simulink model "I_Control_Dcmotor"  (R2022b)
settings: Solver=ode4  StartTime=0.0  StopTime=inf  RelTol=1e-3  EnableMultiTasking=on
libraries: arduinolib x4, arduinosensorlib x1
settings Model: ExtModeTrigDuration=2  Creator=user  LastModifiedBy=user
settings OptimizationCC: EnhancedBackFolding=on  PassReuseOutputArgsAs=Individual arguments  ZeroExternalMemoryAtStartup=off  ZeroInternalMemoryAtStartup=off  MaxStackSize=64  OptimizeBlockOrder=speed  DifferentSizesBufferReuse=on  OptimizationCustomize=off  EfficientTunableParamExpr=on
settings DebuggingCC: ParameterTunabilityLossMsg=error
settings HardwareCC: ProdBitPerInt=16  ProdBitPerPointer=16  ProdBitPerSizeT=16  ProdBitPerPtrDiffT=16  ProdLargestAtomicFloat=None  ProdWordSize=8  ProdHWDeviceType=Atmel->AVR
settings SFSimCC: MATLABDynamicMemAlloc=off
settings RTWCC: Description=Embedded Coder  SystemTargetFile=ert.tlc  HardwareBoard=Arduino Mega 2560  TLCOptions=-aInlineSetEventsForThisBaseRateFcn=TLC_FALSE -aSuppressMultiTaskScheduler=TLC_FALSE -aRateBasedStepFcn=1  TemplateMakefile=ert_default_tmf  Toolchain=Arduino AVR  BuildConfiguration=Faster Runs
settings CodeAppCC: ForceParamTrailComments=on  IgnoreCustomStorageClasses=off  OperatorAnnotations=on  SimulinkDataObjDesc=on  SFDataObjDesc=on  InsertBlockDesc=on
settings ERTTargetCC: SupportContinuousTime=on  SupportVariableSizeSignals=on  ExtModeTransport=3  ExtModeStaticAlloc=on  ExtModeAutomaticAllocSize=off  ExtModeStaticAllocSize=2048  ExtModeMexFile=ext_xcp  ExtModeIntrfLevel=Level2 - Open

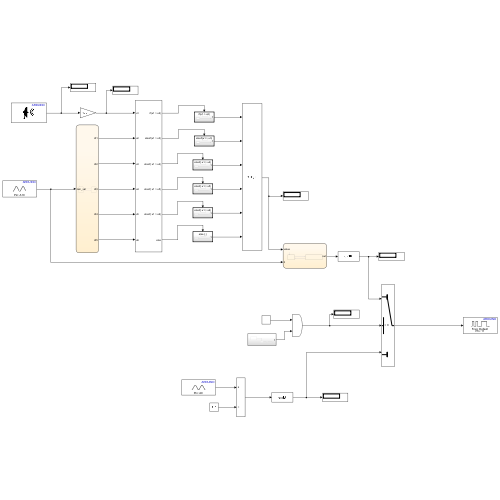
[thumbnail: Simulink's stored preview of the top-level diagram]
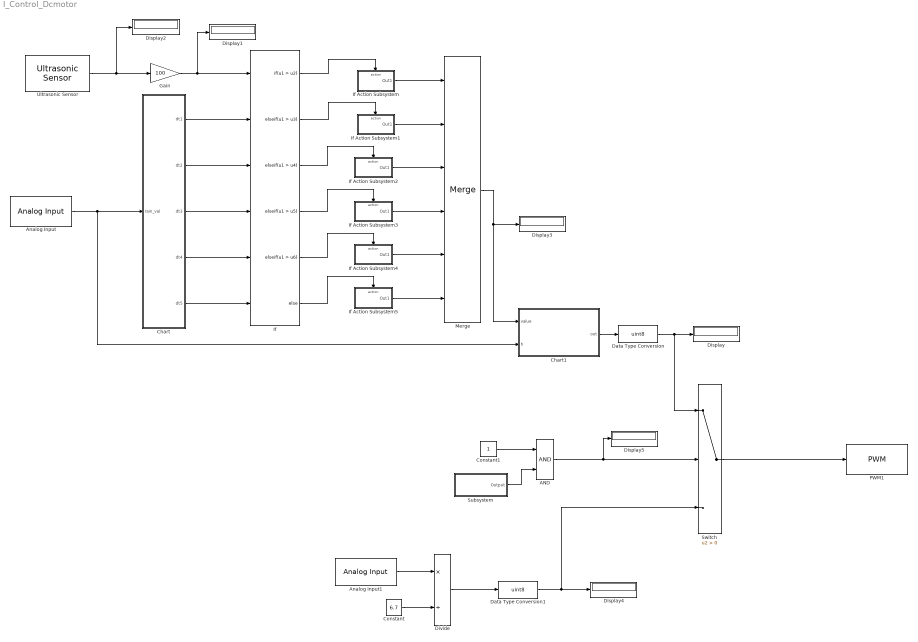
== system I_Control_Dcmotor ==
  AND : Logic  IconShape=distinctive  AllPortsSameDT=off  OutDataTypeStr=boolean
  Analog Input : arduinolib/Analog Input  pinNumber=10  ReadResultsOnly=off  ConversionTriggerSource=Software  ExternalTriggerType=uint32( 0 )  OutputDataType=uint16  EnableConversionCompleteNotify=off  EnableOuputStatus=off  SampleTime=-1  blockPlatform=arduino
  Analog Input1 : arduinolib/Analog Input  pinNumber=0  ReadResultsOnly=off  ConversionTriggerSource=Software  ExternalTriggerType=uint32( 0 )  OutputDataType=uint16  EnableConversionCompleteNotify=off  EnableOuputStatus=off  SampleTime=-1  blockPlatform=arduino
  Chart : Stateflow chart  TreatAsAtomicUnit=on
  Chart1 : Stateflow chart  TreatAsAtomicUnit=on
      settings: PortSchema="{\"entries\":[{\"content\":{\"sides\":[{\"content\":{\"connectorIds\":[\"In2\",\"In1\"]},\"type\":\"ConnectorPlacement.EquallySpacedRectSide\",\"uuid\":\"b8bc21d1-4b9f-4189-a812-b41a4c5af9e6\"},{\"content\":{\"connectorIds\":[\"Out1\"],\"side\":\"RIGHT\"},\"type\":\"ConnectorPlacement.EquallySpacedRectSide\",\"uuid\":\"2c64dce3-08c2-4220-8c60-db9aba55cb61\"},{\"content\":{\"connectorIds\":[],\"side\":\"TOP\"},\"type\":\"ConnectorPlacement.EquallySpacedRectSide\",\"uuid\":\"e1e14768-a3b4-4969-ba09-2d2b4c878f0a\"}]},\"type\":\"ConnectorPlacement.EquallySpacedConnector\",\"uuid\":\"33700ad2-0727-43da-b85e-9713a6dc3065\"}],\"packageUris\":[\"http://schema.mathworks.com/mf0/Connector/R2020b\"],\"version\":\"1.0\"}"
  Constant : Constant  Value=6.7
  Constant1 : Constant
  Data Type Conversion : DataTypeConversion  OutDataTypeStr=uint8  SaturateOnIntegerOverflow=off  RndMeth=Floor
  Data Type Conversion1 : DataTypeConversion  OutDataTypeStr=uint8  SaturateOnIntegerOverflow=off  RndMeth=Floor
  Display{,1..5} (6 alike) : Display
  Divide : Product  Inputs=*/
  Gain : Gain  Gain=100
  If : If  NumInputs=6  IfExpression=u1 > u2  ElseIfExpressions=u1 > u3, u1 > u4, u1 > u5, u1 > u6
  If Action Subsystem : Subsystem  TreatAsAtomicUnit=on
  If Action Subsystem1 : Subsystem  TreatAsAtomicUnit=on
  If Action Subsystem2 : Subsystem  TreatAsAtomicUnit=on
  If Action Subsystem3 : Subsystem  TreatAsAtomicUnit=on
  If Action Subsystem4 : Subsystem  TreatAsAtomicUnit=on
  If Action Subsystem5 : Subsystem  TreatAsAtomicUnit=on
  Merge : Merge  Inputs=6
  PWM1 : arduinolib/PWM  pinNumber=11  frequencyType=Default  desiredFrequency=490.2  achievableFrequency=490.2
  Subsystem : Subsystem
  Switch : Switch  Criteria=u2 > Threshold  SaturateOnIntegerOverflow=off  InputSameDT=off
  Ultrasonic Sensor : arduinosensorlib/Ultrasonic Sensor  NumSignalPins=2  TrigPin=50  EchoPin=51  SignalPin=3  SampleTime_=0.1  blockPlatform=ARDUINO
  wires:
  Ultrasonic Sensor/1 -> Display2/1, Gain/1
  Chart/1(dt1) -> If/2
  Chart/2(dt2) -> If/3
  Chart/3(dt3) -> If/4
  Chart/5(dt5) -> If/6
  Chart/4(dt4) -> If/5
  If Action Subsystem/1(Out1) -> Merge/1
  Gain/1 -> Display1/1, If/1
  If/2 -> If Action Subsystem1/Action
  If/3 -> If Action Subsystem2/Action
  If/4 -> If Action Subsystem3/Action
  If/5 -> If Action Subsystem4/Action
  If/6 -> If Action Subsystem5/Action
  If/1 -> If Action Subsystem/Action
  If Action Subsystem1/1(Out1) -> Merge/2
  If Action Subsystem2/1(Out1) -> Merge/3
  If Action Subsystem3/1(Out1) -> Merge/4
  If Action Subsystem4/1(Out1) -> Merge/5
  If Action Subsystem5/1(Out1) -> Merge/6
  Merge/1 -> Display3/1, Chart1/2(value)
  Analog Input/1 -> Chart1/1(h), Chart/1(rain_val)
  Chart1/1(out) -> Data Type Conversion/1
  Data Type Conversion/1 -> Switch/1, Display/1
  AND/1 -> Display5/1, Switch/2
  Divide/1 -> Data Type Conversion1/1
  Switch/1 -> PWM1/1
  Constant1/1 -> AND/1
  Data Type Conversion1/1 -> Switch/3, Display4/1
  Constant/1 -> Divide/2
  Subsystem/1(Output) -> AND/2
  Analog Input1/1 -> Divide/1

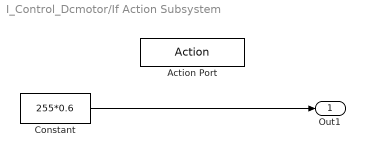
== system I_Control_Dcmotor/If Action Subsystem ==
  Action Port : ActionPort  ActionPortLabel=if(u1 > u2)
  Constant : Constant  Value=255*0.6
  Out1 : Outport
  wires:
  Constant/1 -> Out1/1

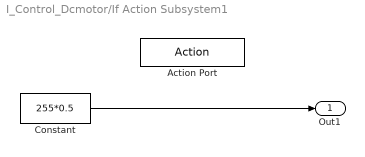
== system I_Control_Dcmotor/If Action Subsystem1 ==
  Action Port : ActionPort  ActionPortLabel=elseif(u1 > u3)
  Constant : Constant  Value=255*0.5
  Out1 : Outport
  wires:
  Constant/1 -> Out1/1

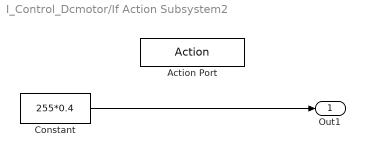
== system I_Control_Dcmotor/If Action Subsystem2 ==
  Action Port : ActionPort  ActionPortLabel=elseif( u1 > u4)
  Constant : Constant  Value=255*0.4
  Out1 : Outport
  wires:
  Constant/1 -> Out1/1

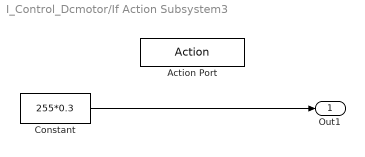
== system I_Control_Dcmotor/If Action Subsystem3 ==
  Action Port : ActionPort  ActionPortLabel=elseif( u1 > u5)
  Constant : Constant  Value=255*0.3
  Out1 : Outport
  wires:
  Constant/1 -> Out1/1

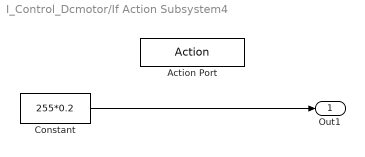
== system I_Control_Dcmotor/If Action Subsystem4 ==
  Action Port : ActionPort  ActionPortLabel=elseif( u1 > u6)
  Constant : Constant  Value=255*0.2
  Out1 : Outport
  wires:
  Constant/1 -> Out1/1

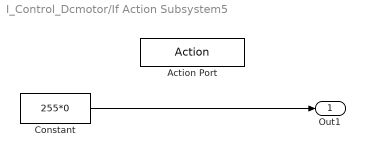
== system I_Control_Dcmotor/If Action Subsystem5 ==
  Action Port : ActionPort  ActionPortLabel=else
  Constant : Constant  Value=255*0
  Out1 : Outport
  wires:
  Constant/1 -> Out1/1

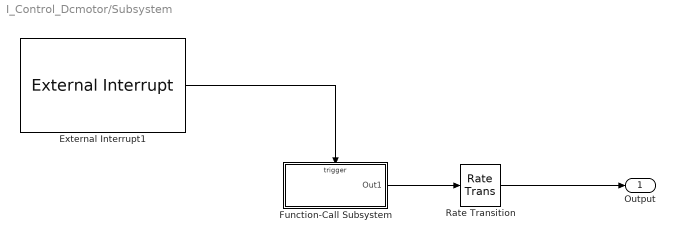
== system I_Control_Dcmotor/Subsystem ==
  External Interrupt1 : arduinolib/External Interrupt  Pin=2  PullUp=off  Mode=FALLING  InterruptSimulationInput=off
  Function-Call Subsystem : Subsystem  TreatAsAtomicUnit=on
  Rate Transition : RateTransition  Deterministic=off
  Output : Outport
  wires:
  Function-Call Subsystem/1(Out1) -> Rate Transition/1
  External Interrupt1/1 -> Function-Call Subsystem/Trigger
  Rate Transition/1 -> Output/1

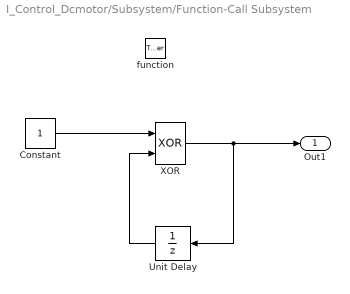
== system I_Control_Dcmotor/Subsystem/Function-Call Subsystem ==
  function : TriggerPort  TriggerType=function-call  VariantControl=(inherit)
  Constant : Constant
  Unit Delay : UnitDelay  InitialCondition=1  SampleTime=-1  HasFrameUpgradeWarning=on
  XOR : Logic  Operator=XOR  IconShape=distinctive  AllPortsSameDT=off  OutDataTypeStr=boolean
  Out1 : Outport
  wires:
  Constant/1 -> XOR/1
  XOR/1 -> Unit Delay/1, Out1/1
  Unit Delay/1 -> XOR/2

== stateflow chart I_Control_Dcmotor/Chart1 ==
  state not_rain
    out = value
  state rain
    out = value - (((255*0.6) - value) *0.5)
  (default) -> not_rain
  not_rain -> rain : [h<=800]
  rain -> not_rain : [h>800]
  data: h input; value input; out output

== stateflow chart I_Control_Dcmotor/Chart ==
  state Non_rain
    dt1 = 50
    dt2 = 40
    dt3 = 30
    dt4 = 20
    dt5 = 10
  state Rain
    dt1=55
    dt2=45
    dt3=35
    dt4=25
    dt5=15
  (default) -> Non_rain
  Rain -> Non_rain : [rain_val > 800]
  Non_rain -> Rain : [rain_val <= 800]
  data: dt1 output; dt2 output; dt3 output; dt4 output; dt5 output; rain_val input
